simulink model "ass2"  (R2018a)
settings: Solver=VariableStepAuto  StartTime=0.0  StopTime=10.0  RelTol=1e-3
settings Model: Creator=22121100  LastModifiedBy=22121100

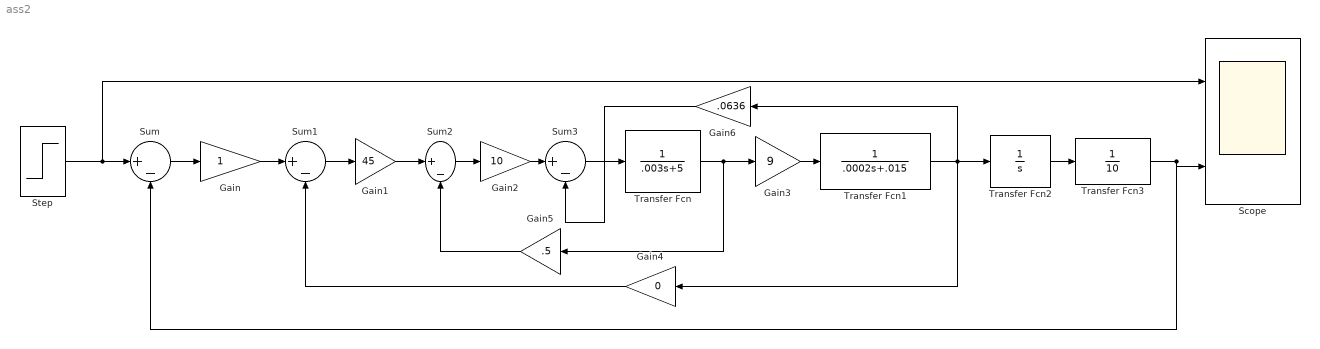
== system ass2 ==
  Gain : Gain
  Gain1 : Gain  Gain=45
  Gain2 : Gain  Gain=10
  Gain3 : Gain  Gain=9
  Gain4 : Gain  Gain=0
  Gain5 : Gain  Gain=.5
  Gain6 : Gain  Gain=.0636
  Scope : Scope  NumInputPorts=2
  Step : Step  SampleTime=0
  Sum{,1..3} (4 alike) : Sum  Inputs=|+-
  Transfer Fcn : TransferFcn  Denominator=[.003 5]
  Transfer Fcn1 : TransferFcn  Denominator=[.0002 .015]
  Transfer Fcn2 : TransferFcn  Denominator=[1 0]
  Transfer Fcn3 : TransferFcn  Denominator=[0 10]
  wires:
  Step/1 -> Sum/1, Scope/1
  Sum/1 -> Gain/1
  Gain1/1 -> Sum2/1
  Gain/1 -> Sum1/1
  Sum1/1 -> Gain1/1
  Sum2/1 -> Gain2/1
  Transfer Fcn/1 -> Gain5/1, Gain3/1
  Gain3/1 -> Transfer Fcn1/1
  Transfer Fcn1/1 -> Gain4/1, Transfer Fcn2/1, Gain6/1
  Transfer Fcn2/1 -> Transfer Fcn3/1
  Gain5/1 -> Sum2/2
  Gain4/1 -> Sum1/2
  Transfer Fcn3/1 -> Sum/2, Scope/2
  Gain2/1 -> Sum3/1
  Sum3/1 -> Transfer Fcn/1
  Gain6/1 -> Sum3/2
